simulink model "Simple_Model_Packaging_1_1"  (R2022b)
settings: Solver=VariableStepAuto  StartTime=0.0  StopTime=0.001  RelTol=1e-3
InitFcn:
  | Parameter_Initialize_1
undefined symbols (not defined in the file or in its folder): gcbh, magnitude, model, rcfiltgaincompat, rsgenpoly
libraries: commdigbbndpm3 x3, commsynccomp2 x3, commdigbbndam3 x2, commdigbbndfm2 x2, simulink x2, commblkcod2 x1, commfilt2 x1, commrandsrc3 x1
settings Model: Creator=89778  LastModifiedBy=z0y

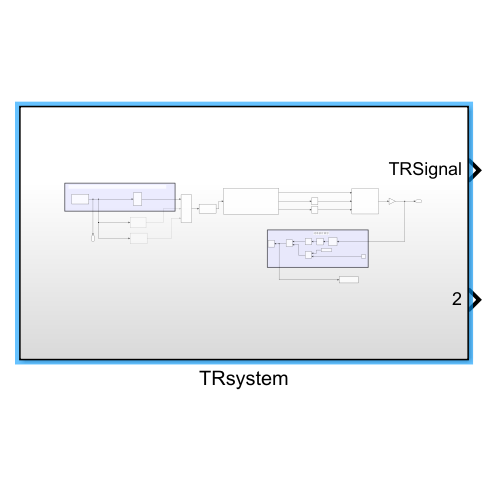
[thumbnail: Simulink's stored preview of the top-level diagram]
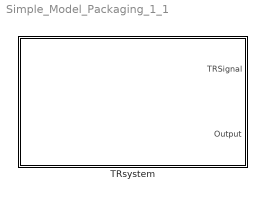
== system Simple_Model_Packaging_1_1 ==
  TRsystem : Subsystem

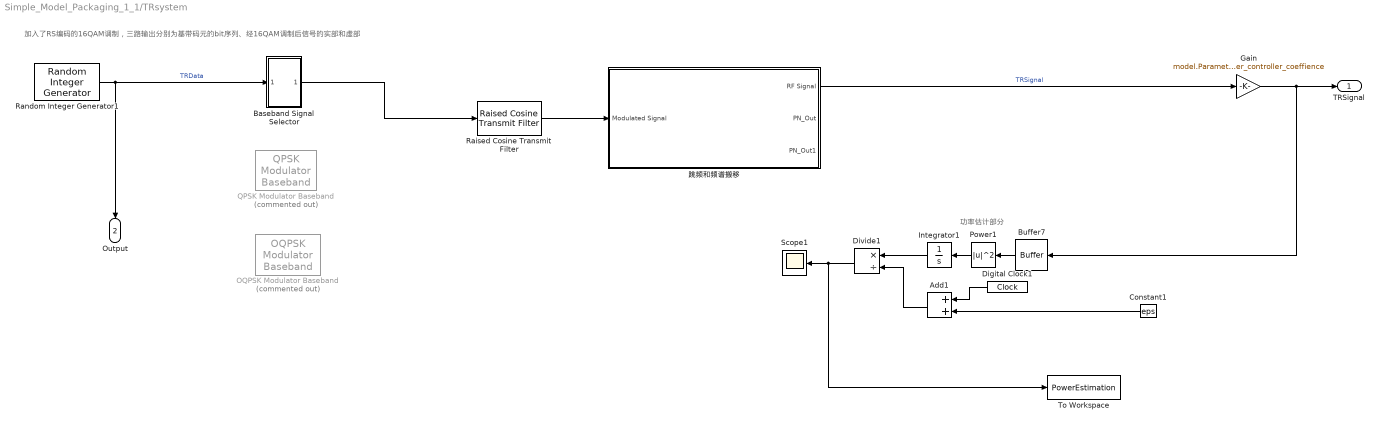
== system Simple_Model_Packaging_1_1/TRsystem ==
  note: 功率估计部分
  note: 加入了RS编码的16QAM调制，三路输出分别为基带码元的bit序列、经16QAM调制后信号的实部和虚部
  Add1 : Sum
  Baseband Signal Selector : Subsystem
  Buffer7 : Buffer  N=1  OutputFrames=off
  Constant1 : Constant  Value=eps  SampleTime=model.Parameters.TR.system_frame_speed
  Digital Clock1 : DigitalClock  SampleTime=model.Parameters.TR.system_frame_speed
  Divide1 : Product  Inputs=*/
  Gain : Gain  Gain=model.Parameters.TR.communication_sig_power_controller_coeffience
  Integrator1 : Integrator
  OQPSK Modulator Baseband : commdigbbndpm3/OQPSK Modulator Baseband  Commented=on  InType=Integer  Ph=0  Mapping=Gray  pulseShape=Half sine  num=[0.7071, 0.7071]  rolloff=0.2  filterSpan=10  sps=2  RateOptions=Enforce single-rate processing  outDtype=double
  Power1 : Math  Operator=magnitude^2
  QPSK Modulator Baseband : commdigbbndpm3/QPSK Modulator Baseband  Commented=on  InType=Integer  Enc=Gray  Ph=pi/4  outDtype=double  outWordLen=16  outUDDataType=sfix(16)  outFracLenMode=Best precision  outFracLen=15  outDataTypeStr=double  outLastDataTypeStr=double
  Raised Cosine Transmit Filter : commfilt2/Raised Cosine Transmit Filter  filtType=Square root  R=model.Parameters.TR.Raised_Cosine_Transmit_Filter.Rolloff_factor  filtSpan=model.Parameters.TR.Raised_Cosine_Transmit_Filter.Filter_span_in_symbols  N=model.Parameters.TR.Raised_Cosine_Transmit_Filter.Output_samples_per_symbol  filterGain=rcfiltgaincompat(gcbh)  InputProcessing=Columns as channels (frame based)  RateOptions=Enforce single-rate processing  framing=Mute  checkCoeff=off  variableName=rcTxFilt  checkGain=Normalized  sampMode=Mute  saveAsFlag=0  currentFiltSpan=10  D=(10)/2  launchFVT=on  roundingMode=Floor  overflowMode=off  coeffDataTypeStr=Inherit: Same word length as input  coeffMin=[]  coeffMax=[]  coeffLastDataTypeStr=Inherit: Same word length as input  outputDataTypeStr=Inherit: Same as accumulator  outputMin=[]  outputMax=[]  outputLastDataTypeStr=Inherit: Same as accumulator
  Random Integer Generator1 : commrandsrc3/Random Integer Generator  SetSize=model.Parameters.TR.Random_Integer_Generator.SetSize  SeedSource=Auto  Seed=4  SampleTime=model.Parameters.TR.Random_Integer_Generator.Random_Sample_Time  SamplesPerFrame=model.Parameters.TR.Random_Integer_Generator.Samples_per_frame  OutputDataType=double  SimulateUsing=Interpreted execution
  Scope1 : Scope
  To Workspace : ToWorkspace  VariableName=PowerEstimation  SaveFormat=Timeseries  SampleTime=-1
  跳频和频谱搬移 : Subsystem
  TRSignal : Outport
  Output : Outport  Port=2
  wires:
  Random Integer Generator1/1 -> Output/1, Baseband Signal Selector/1(In1)  "TRData"
  Raised Cosine Transmit Filter/1 -> 跳频和频谱搬移/1(Modulated Signal)
  Add1/1 -> Divide1/2
  Digital Clock1/1 -> Add1/1
  Divide1/1 -> To Workspace/1, Scope1/1
  Integrator1/1 -> Divide1/1
  Constant1/1 -> Add1/2
  跳频和频谱搬移/1(RF Signal) -> Gain/1  "TRSignal"
  Buffer7/1 -> Power1/1
  Power1/1 -> Integrator1/1
  Gain/1 -> Buffer7/1, TRSignal/1
  Baseband Signal Selector/1(Out1) -> Raised Cosine Transmit Filter/1

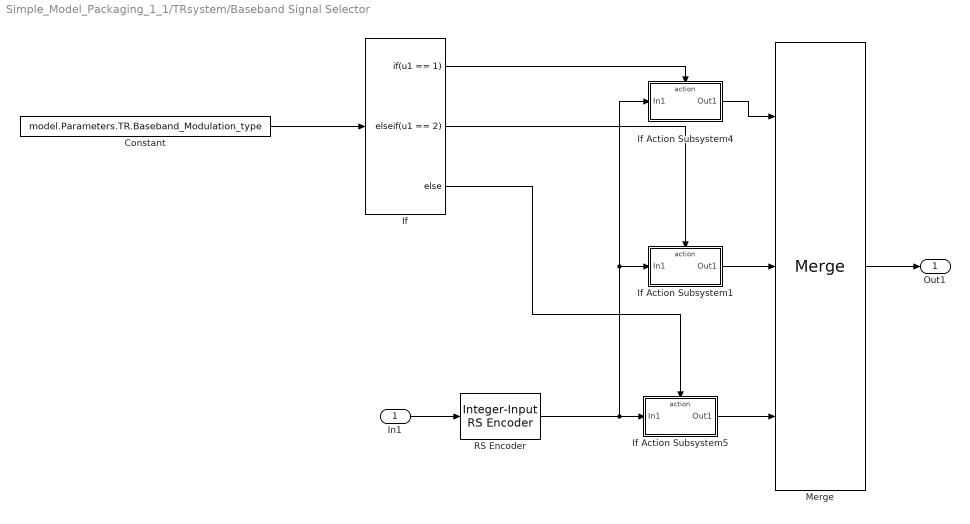
== system Simple_Model_Packaging_1_1/TRsystem/Baseband Signal Selector ==
  In1 : Inport
  Constant : Constant  Value=model.Parameters.TR.Baseband_Modulation_type
  If : If  IfExpression=u1 == 1  ElseIfExpressions=u1 == 2
  If Action Subsystem1 : Subsystem  TreatAsAtomicUnit=on
  If Action Subsystem4 : Subsystem  TreatAsAtomicUnit=on
  If Action Subsystem5 : Subsystem  TreatAsAtomicUnit=on
  Merge : Merge  Inputs=3
  RS Encoder : commblkcod2/Integer-Input RS Encoder  n=model.Parameters.TR.RS_Encoder.Codeword_Length  k=model.Parameters.TR.RS_Encoder.Message_Length  specShortening=off  shortenedK=3  specGenPoly=off  genPoly=rsgenpoly(7,3)  specPrimPoly=off  prPoly=[1 0 1 1]  specPuncture=off  punctVec=[ones(2,1); zeros(2,1)]
  Out1 : Outport
  wires:
  In1/1 -> RS Encoder/1
  If Action Subsystem5/1(Out1) -> Merge/3
  Constant/1 -> If/1
  Merge/1 -> Out1/1
  If/3 -> If Action Subsystem5/Action
  If/1 -> If Action Subsystem4/Action
  If/2 -> If Action Subsystem1/Action
  If Action Subsystem1/1(Out1) -> Merge/2
  If Action Subsystem4/1(Out1) -> Merge/1
  RS Encoder/1 -> If Action Subsystem4/1(In1), If Action Subsystem1/1(In1), If Action Subsystem5/1(In1)

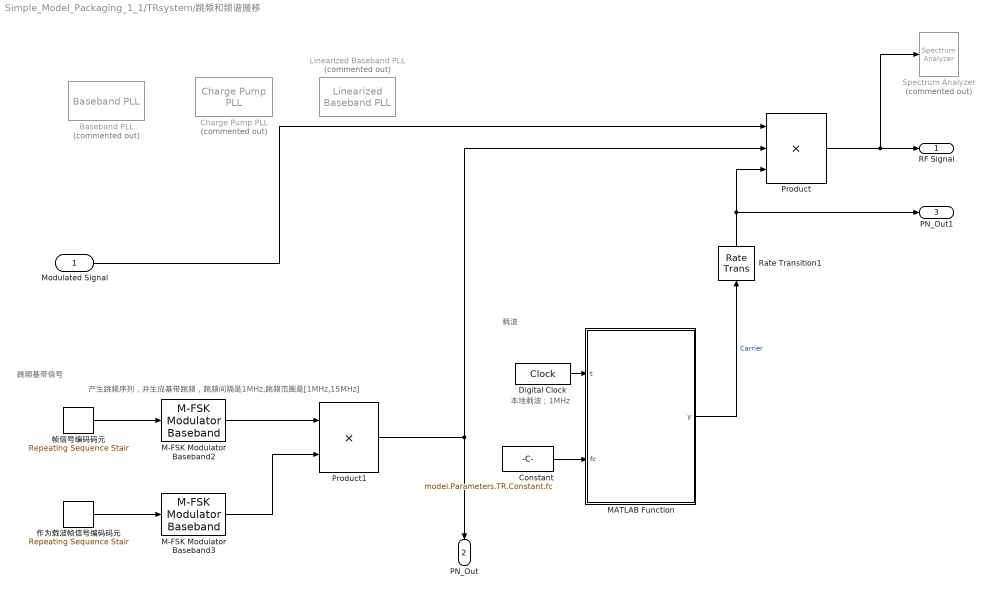
== system Simple_Model_Packaging_1_1/TRsystem/跳频和频谱搬移 ==
  note: 本地载波 ; 1MHz
  note: 跳频基带信号
  note: 载波
  note: 产生跳频序列，并生成基带跳频，跳频间隔是1MHz,跳频范围是[1MHz,15MHz]
  Modulated Signal : Inport
  Baseband PLL : commsynccomp2/Baseband PLL  Commented=on  Fn="[3.0002  0  40002]"  Fd="[1   67.46   2270.9   40002]"  Kvco=1
  Charge Pump PLL : commsynccomp2/Charge Pump PLL  Commented=on  Fn="[3.0002  0  40002]"  Fd="[1   67.46   2270.9   40002]"  Kvco=1  Fc=100  Ph=0  Ac=1
  Constant : Constant  Value=model.Parameters.TR.Constant.fc
  Digital Clock : DigitalClock  SampleTime=model.Parameters.TR.Digital_Clock.fc_Ts
  Linearized Baseband PLL : commsynccomp2/Linearized Baseband PLL  Commented=on  Fn="[3.0002  0  40002]"  Fd="[1   67.46   2270.9   40002]"  Kvco=1
  M-FSK Modulator Baseband2 : commdigbbndfm2/M-FSK Modulator Baseband  M=model.Parameters.TR.M_FSK_Modulator_Baseband1.M_ary_number  InType=Integer  Enc=Binary  freqSep=model.Parameters.TR.M_FSK_Modulator_Baseband1.Frequency_separation  phaseType=Continuous  numSamp=model.Parameters.TR.M_FSK_Modulator_Baseband1.Samples_per_symbol  RateOptions=Enforce single-rate processing  outDataType=double
  M-FSK Modulator Baseband3 : commdigbbndfm2/M-FSK Modulator Baseband  M=model.Parameters.TR.M_FSK_Modulator_Baseband1.M_ary_number  InType=Integer  Enc=Binary  freqSep=model.Parameters.TR.M_FSK_Modulator_Baseband1.Frequency_separation  phaseType=Continuous  numSamp=model.Parameters.TR.M_FSK_Modulator_Baseband1.Samples_per_symbol  RateOptions=Enforce single-rate processing  outDataType=double
  MATLAB Function : MATLAB Function  TreatAsAtomicUnit=on
  Product : Product  Inputs=3
  Product1 : Product
  Rate Transition1 : RateTransition
  Spectrum Analyzer : SpectrumAnalyzer  Commented=on
  作为载波帧信号编码码元 : simulink/Sources/Repeating Sequence Stair  OutValues=[model.Parameters.TR.M_FSK_Modulator_Baseband1.M_ary_number-1]  tsamp=model.Parameters.frame_of_hopping_Sample_time  OutMin=[]  OutMax=[]  OutDataTypeStr=double  OutputDataTypeScalingMode=double  OutDataType=fixdt(0,8)  ConRadixGroup=Best Precision: Vector-wise  OutScaling=2^-12
  帧信号编码码元 : simulink/Sources/Repeating Sequence Stair  OutValues=model.parameter.frame_of_hopping_output_vector  tsamp=model.Parameters.frame_of_hopping_Sample_time  OutMin=[]  OutMax=[]  OutDataTypeStr=double  OutputDataTypeScalingMode=double  OutDataType=fixdt(0,8)  ConRadixGroup=Best Precision: Vector-wise  OutScaling=2^-12
  RF Signal : Outport
  PN_Out : Outport  Port=2
  PN_Out1 : Outport  Port=3
  wires:
  Modulated Signal/1 -> Product/1
  Product/1 -> Spectrum Analyzer/1, RF Signal/1
  Digital Clock/1 -> MATLAB Function/1(t)
  Product1/1 -> Product/2, PN_Out/1
  MATLAB Function/1(y) -> Rate Transition1/1  "Carrier"
  Rate Transition1/1 -> Product/3, PN_Out1/1
  Constant/1 -> MATLAB Function/2(fc)
  作为载波帧信号编码码元/1 -> M-FSK Modulator Baseband3/1
  M-FSK Modulator Baseband2/1 -> Product1/1
  帧信号编码码元/1 -> M-FSK Modulator Baseband2/1
  M-FSK Modulator Baseband3/1 -> Product1/2

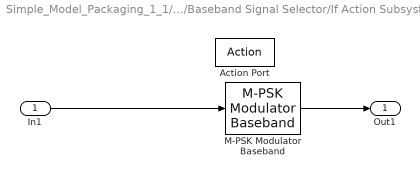
== system Simple_Model_Packaging_1_1/TRsystem/Baseband Signal Selector/If Action Subsystem1 ==
  In1 : Inport
  Action Port : ActionPort  ActionPortLabel=elseif(u1 == 2)
  M-PSK Modulator Baseband : commdigbbndpm3/M-PSK Modulator Baseband  M=model.Parameters.TR.Rectangular_QAM_Modulator_Baseband.M_Number  InType=Integer  Enc=Gray  Mapping=[0:7]  Ph=0  outDtype=double  outWordLen=16  outUDDataType=sfix(16)  outFracLenMode=Best precision  outFracLen=15  outDataTypeStr=double  outLastDataTypeStr=double
  Out1 : Outport
  wires:
  M-PSK Modulator Baseband/1 -> Out1/1
  In1/1 -> M-PSK Modulator Baseband/1

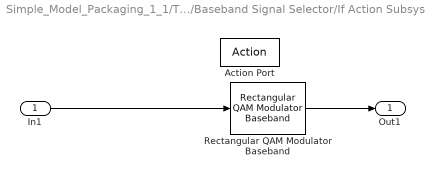
== system Simple_Model_Packaging_1_1/TRsystem/Baseband Signal Selector/If Action Subsystem4 ==
  In1 : Inport
  Action Port : ActionPort  ActionPortLabel=if(u1 == 1)
  Rectangular QAM Modulator Baseband : commdigbbndam3/Rectangular QAM Modulator Baseband  M=model.Parameters.TR.Rectangular_QAM_Modulator_Baseband.M_Number  InType=Integer  Enc=Gray  Mapping=[0:15]  PowType=Min. distance between symbols  MinDist=model.Parameters.TR.Rectangular_QAM_Modulator_Baseband.Minimum_distance  AvgPow=1  PeakPow=1  Ph=0  outDtype=double  outWordLen=16  outUDDataType=sfix(16)  outFracLenMode=Best precision  outFracLen=15  outDataTypeStr=double  outLastDataTypeStr=double
      settings: LibrarySourceBlock=|
      | commhdldigbbndam/Rectangular QAM
      | Modulator
      | Baseband
  Out1 : Outport
  wires:
  Rectangular QAM Modulator Baseband/1 -> Out1/1
  In1/1 -> Rectangular QAM Modulator Baseband/1

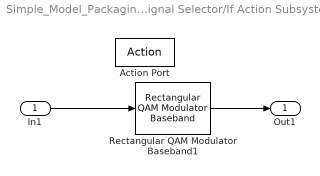
== system Simple_Model_Packaging_1_1/TRsystem/Baseband Signal Selector/If Action Subsystem5 ==
  In1 : Inport
  Action Port : ActionPort  ActionPortLabel=else
  Rectangular QAM Modulator Baseband1 : commdigbbndam3/Rectangular QAM Modulator Baseband  M=model.Parameters.TR.Rectangular_QAM_Modulator_Baseband.M_Number  InType=Integer  Enc=Gray  Mapping=[0:15]  PowType=Min. distance between symbols  MinDist=model.Parameters.TR.Rectangular_QAM_Modulator_Baseband.Minimum_distance  AvgPow=1  PeakPow=1  Ph=0  outDtype=double  outWordLen=16  outUDDataType=sfix(16)  outFracLenMode=Best precision  outFracLen=15  outDataTypeStr=double  outLastDataTypeStr=double
      settings: LibrarySourceBlock=|
      | commhdldigbbndam/Rectangular QAM
      | Modulator
      | Baseband
  Out1 : Outport
  wires:
  In1/1 -> Rectangular QAM Modulator Baseband1/1
  Rectangular QAM Modulator Baseband1/1 -> Out1/1

== matlab function Simple_Model_Packaging_1_1/TRsystem/跳频和频谱搬移/MATLAB Function ==
  data: y output; t input; fc input
function y = fcn(t,fc)
%     fs = 40e6;
%     Ts = 1/fs;
%     t = 0:Ts:0.002;
%     fc = 1e6;
    y = exp(1i*2*pi*fc*t);

end
